simulink model "SWC_APS_type"  (R2021b)
settings: Solver=FixedStepDiscrete  StartTime=0.0  StopTime=10.0  RelTol=1e-3
settings Model: DataDictionary=APPTypes.sldd  Creator=FVT23010  LastModifiedBy=FVT23010
settings DataIOCC: SaveFormat=StructureWithTime
settings OptimizationCC: DefaultParameterBehavior=Inlined  EnhancedBackFolding=on  PassReuseOutputArgsAs=Individual arguments  ZeroExternalMemoryAtStartup=off  ZeroInternalMemoryAtStartup=off  OptimizeBlockOrder=speed  DifferentSizesBufferReuse=on  OptimizationCustomize=off  EfficientTunableParamExpr=on
settings DebuggingCC: ParameterTunabilityLossMsg=error
settings SFSimCC: MATLABDynamicMemAlloc=off
settings RTWCC: Description=AUTOSAR  SystemTargetFile=autosar.tlc  GenCodeOnly=on  TemplateMakefile=ert_default_tmf
settings CodeAppCC: ForceParamTrailComments=on  IgnoreCustomStorageClasses=off  OperatorAnnotations=on  SimulinkDataObjDesc=on  SFDataObjDesc=on  InsertBlockDesc=on
settings STFCustomTargetCC: TargetLangStandard=C99 (ISO)  MultiwordLength=256  ParMdlRefBuildCompliant=on  CompOptLevelCompliant=on  IncludeMdlTerminateFcn=off  CombineOutputUpdateFcns=on  SuppressErrorStatus=on  ERTCustomFileBanners=on  SupportNonFinite=off  SupportComplex=off  SupportContinuousTime=off  SupportNonInlinedSFcns=off  RemoveResetFunc=on  MATLABClassNameForMDSCustomization=Simulink.SoftwareTarget.ERTCustomization  AutosarCompliant=on  GRTInterface=off  UseToolchainInfoCompliant=on  LookupTableObjectStructAxisOrder=2,1,3,4,...  LUTObjectStructOrderEvenSpacing=Size,Table,Breakpoints  SystemTargetFile=autosar.tlc
settings ERTTargetCC: TargetLangStandard=C99 (ISO)  ConcurrentExecutionCompliant=off  IncludeMdlTerminateFcn=off  SuppressErrorStatus=on  SupportNonFinite=off  SupportComplex=off  ModelStepFunctionPrototypeControlCompliant=off  CPPClassGenCompliant=off  AutosarCompliant=on  LookupTableObjectStructAxisOrder=2,1,3,4,...  LUTObjectStructOrderEvenSpacing=Size,Table,Breakpoints  InlinedParameterPlacement=NonHierarchical  ERTCustomFileTemplate=example_file_process.tlc

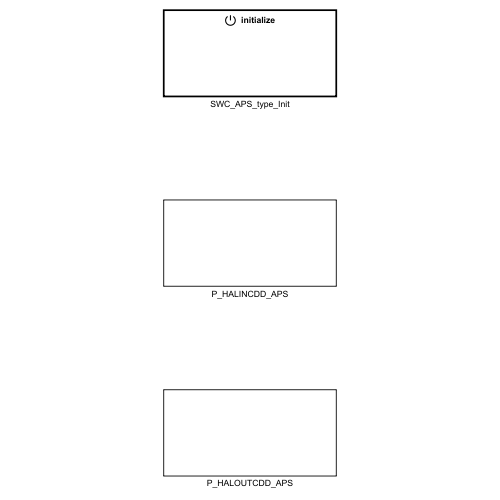
[thumbnail: Simulink's stored preview of the top-level diagram]
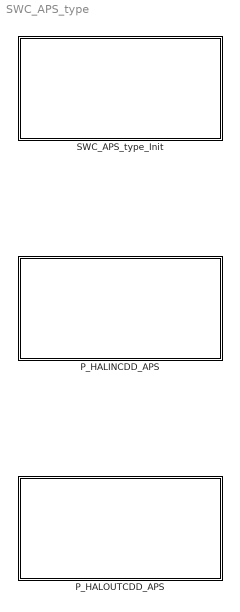
== system SWC_APS_type ==
  P_HALINCDD_APS : Subsystem
  P_HALOUTCDD_APS : Subsystem
  SWC_APS_type_Init : Subsystem

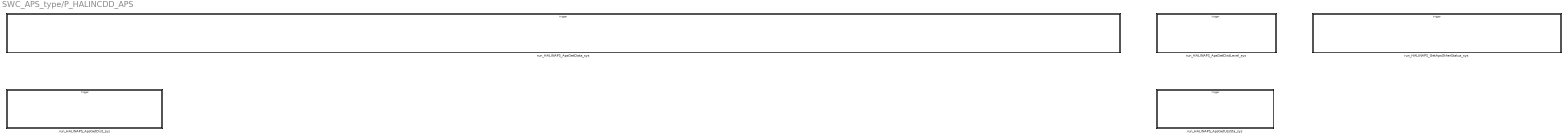
== system SWC_APS_type/P_HALINCDD_APS ==
  run_HALINAPS_ApsGetData_sys : Subsystem
  run_HALINAPS_ApsGetDistLevel_sys : Subsystem
  run_HALINAPS_ApsGetDist_sys : Subsystem
  run_HALINAPS_ApsGetUssSta_sys : Subsystem
  run_HALINAPS_GetApsOtherStatus_sys : Subsystem

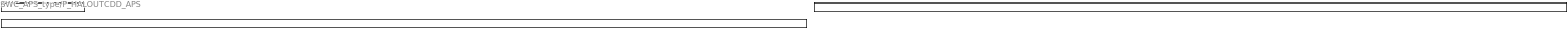
== system SWC_APS_type/P_HALOUTCDD_APS ==
  run_HALOUTAPS_ApsOutput_sys : Subsystem
  run_HALOUTAPS_ApsSetData_sys : Subsystem
  run_HALOUTAPS_ApsSetTimeout_sys : Subsystem

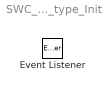
== system SWC_APS_type/SWC_APS_type_Init ==
  Event Listener : EventListener  EventName=reset

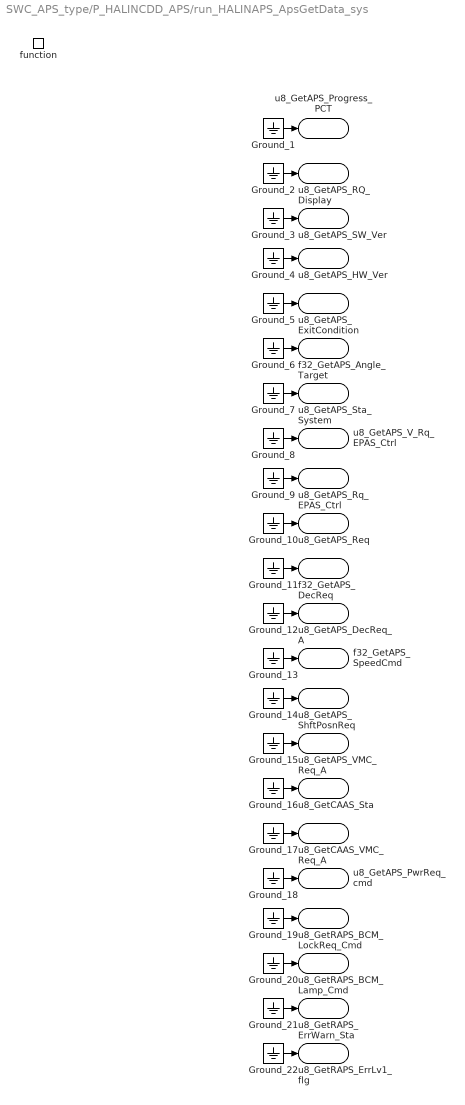
== system SWC_APS_type/P_HALINCDD_APS/run_HALINAPS_ApsGetData_sys ==
  function : TriggerPort  TriggerType=function-call  IsSimulinkFunction=on  FunctionName=run_HALINAPS_ApsGetData  VariantControl=(inherit)
  Ground_{1..22} (22 alike) : Ground
  u8_GetAPS_Progress_PCT : ArgOut  OutDataTypeStr=uint8  ArgumentName=u8_GetAPS_Progress_PCT
  u8_GetAPS_RQ_Display : ArgOut  Port=2  OutDataTypeStr=uint8  ArgumentName=u8_GetAPS_RQ_Display
  u8_GetAPS_SW_Ver : ArgOut  Port=3  OutDataTypeStr=uint8  ArgumentName=u8_GetAPS_SW_Ver
  u8_GetAPS_HW_Ver : ArgOut  Port=4  OutDataTypeStr=uint8  ArgumentName=u8_GetAPS_HW_Ver
  u8_GetAPS_ExitCondition : ArgOut  Port=5  OutDataTypeStr=uint8  ArgumentName=u8_GetAPS_ExitCondition
  f32_GetAPS_Angle_Target : ArgOut  Port=6  OutDataTypeStr=single  ArgumentName=f32_GetAPS_Angle_Target
  u8_GetAPS_Sta_System : ArgOut  Port=7  OutDataTypeStr=uint8  ArgumentName=u8_GetAPS_Sta_System
  u8_GetAPS_V_Rq_EPAS_Ctrl : ArgOut  Port=8  OutDataTypeStr=uint8  ArgumentName=u8_GetAPS_V_Rq_EPAS_Ctrl
  u8_GetAPS_Rq_EPAS_Ctrl : ArgOut  Port=9  OutDataTypeStr=uint8  ArgumentName=u8_GetAPS_Rq_EPAS_Ctrl
  u8_GetAPS_Req : ArgOut  Port=10  OutDataTypeStr=uint8  ArgumentName=u8_GetAPS_Req
  f32_GetAPS_DecReq : ArgOut  Port=11  OutDataTypeStr=single  ArgumentName=f32_GetAPS_DecReq
  u8_GetAPS_DecReq_A : ArgOut  Port=12  OutDataTypeStr=uint8  ArgumentName=u8_GetAPS_DecReq_A
  f32_GetAPS_SpeedCmd : ArgOut  Port=13  OutDataTypeStr=single  ArgumentName=f32_GetAPS_SpeedCmd
  u8_GetAPS_ShftPosnReq : ArgOut  Port=14  OutDataTypeStr=uint8  ArgumentName=u8_GetAPS_ShftPosnReq
  u8_GetAPS_VMC_Req_A : ArgOut  Port=15  OutDataTypeStr=uint8  ArgumentName=u8_GetAPS_VMC_Req_A
  u8_GetCAAS_Sta : ArgOut  Port=16  OutDataTypeStr=uint8  ArgumentName=u8_GetCAAS_Sta
  u8_GetCAAS_VMC_Req_A : ArgOut  Port=17  OutDataTypeStr=uint8  ArgumentName=u8_GetCAAS_VMC_Req_A
  u8_GetAPS_PwrReq_cmd : ArgOut  Port=18  OutDataTypeStr=uint8  ArgumentName=u8_GetAPS_PwrReq_cmd
  u8_GetRAPS_BCM_LockReq_Cmd : ArgOut  Port=19  OutDataTypeStr=uint8  ArgumentName=u8_GetRAPS_BCM_LockReq_Cmd
  u8_GetRAPS_BCM_Lamp_Cmd : ArgOut  Port=20  OutDataTypeStr=uint8  ArgumentName=u8_GetRAPS_BCM_Lamp_Cmd
  u8_GetRAPS_ErrWarn_Sta : ArgOut  Port=21  OutDataTypeStr=uint8  ArgumentName=u8_GetRAPS_ErrWarn_Sta
  u8_GetRAPS_ErrLv1_flg : ArgOut  Port=22  OutDataTypeStr=uint8  ArgumentName=u8_GetRAPS_ErrLv1_flg
  wires:
  Ground_1/1 -> u8_GetAPS_Progress_PCT/1
  Ground_2/1 -> u8_GetAPS_RQ_Display/1
  Ground_3/1 -> u8_GetAPS_SW_Ver/1
  Ground_4/1 -> u8_GetAPS_HW_Ver/1
  Ground_5/1 -> u8_GetAPS_ExitCondition/1
  Ground_6/1 -> f32_GetAPS_Angle_Target/1
  Ground_7/1 -> u8_GetAPS_Sta_System/1
  Ground_8/1 -> u8_GetAPS_V_Rq_EPAS_Ctrl/1
  Ground_9/1 -> u8_GetAPS_Rq_EPAS_Ctrl/1
  Ground_10/1 -> u8_GetAPS_Req/1
  Ground_11/1 -> f32_GetAPS_DecReq/1
  Ground_12/1 -> u8_GetAPS_DecReq_A/1
  Ground_13/1 -> f32_GetAPS_SpeedCmd/1
  Ground_14/1 -> u8_GetAPS_ShftPosnReq/1
  Ground_15/1 -> u8_GetAPS_VMC_Req_A/1
  Ground_16/1 -> u8_GetCAAS_Sta/1
  Ground_17/1 -> u8_GetCAAS_VMC_Req_A/1
  Ground_18/1 -> u8_GetAPS_PwrReq_cmd/1
  Ground_19/1 -> u8_GetRAPS_BCM_LockReq_Cmd/1
  Ground_20/1 -> u8_GetRAPS_BCM_Lamp_Cmd/1
  Ground_21/1 -> u8_GetRAPS_ErrWarn_Sta/1
  Ground_22/1 -> u8_GetRAPS_ErrLv1_flg/1

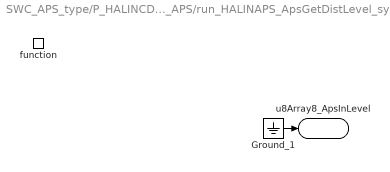
== system SWC_APS_type/P_HALINCDD_APS/run_HALINAPS_ApsGetDistLevel_sys ==
  function : TriggerPort  TriggerType=function-call  IsSimulinkFunction=on  FunctionName=run_HALINAPS_ApsGetDistLevel  VariantControl=(inherit)
  Ground_1 : Ground
  u8Array8_ApsInLevel : ArgOut  OutDataTypeStr=uint8  PortDimensions=8  ArgumentName=u8Array8_ApsInLevel
  wires:
  Ground_1/1 -> u8Array8_ApsInLevel/1

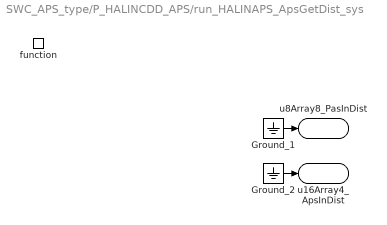
== system SWC_APS_type/P_HALINCDD_APS/run_HALINAPS_ApsGetDist_sys ==
  function : TriggerPort  TriggerType=function-call  IsSimulinkFunction=on  FunctionName=run_HALINAPS_ApsGetDist  VariantControl=(inherit)
  Ground_1 : Ground
  Ground_2 : Ground
  u8Array8_PasInDist : ArgOut  OutDataTypeStr=uint8  PortDimensions=8  ArgumentName=u8Array8_PasInDist
  u16Array4_ApsInDist : ArgOut  Port=2  OutDataTypeStr=uint16  PortDimensions=4  ArgumentName=u16Array4_ApsInDist
  wires:
  Ground_1/1 -> u8Array8_PasInDist/1
  Ground_2/1 -> u16Array4_ApsInDist/1

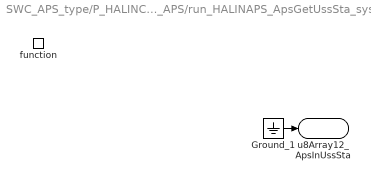
== system SWC_APS_type/P_HALINCDD_APS/run_HALINAPS_ApsGetUssSta_sys ==
  function : TriggerPort  TriggerType=function-call  IsSimulinkFunction=on  FunctionName=run_HALINAPS_ApsGetUssSta  VariantControl=(inherit)
  Ground_1 : Ground
  u8Array12_ApsInUssSta : ArgOut  OutDataTypeStr=uint8  PortDimensions=12  ArgumentName=u8Array12_ApsInUssSta
  wires:
  Ground_1/1 -> u8Array12_ApsInUssSta/1

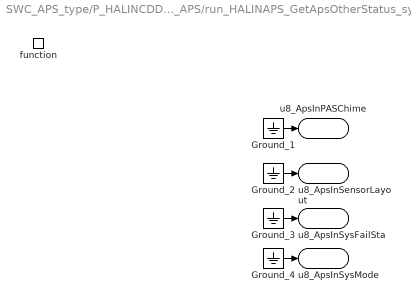
== system SWC_APS_type/P_HALINCDD_APS/run_HALINAPS_GetApsOtherStatus_sys ==
  function : TriggerPort  TriggerType=function-call  IsSimulinkFunction=on  FunctionName=run_HALINAPS_GetApsOtherStatus  VariantControl=(inherit)
  Ground_{1..4} (4 alike) : Ground
  u8_ApsInPASChime : ArgOut  OutDataTypeStr=uint8  ArgumentName=u8_ApsInPASChime
  u8_ApsInSensorLayout : ArgOut  Port=2  OutDataTypeStr=uint8  ArgumentName=u8_ApsInSensorLayout
  u8_ApsInSysFailSta : ArgOut  Port=3  OutDataTypeStr=uint8  ArgumentName=u8_ApsInSysFailSta
  u8_ApsInSysMode : ArgOut  Port=4  OutDataTypeStr=uint8  ArgumentName=u8_ApsInSysMode
  wires:
  Ground_1/1 -> u8_ApsInPASChime/1
  Ground_2/1 -> u8_ApsInSensorLayout/1
  Ground_3/1 -> u8_ApsInSysFailSta/1
  Ground_4/1 -> u8_ApsInSysMode/1

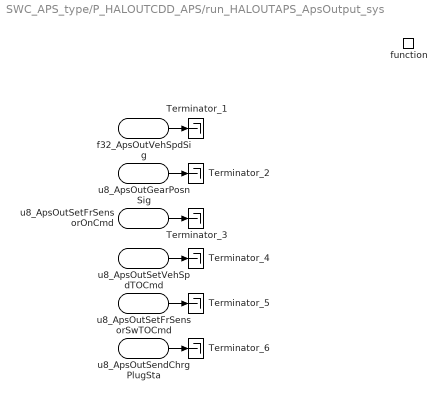
== system SWC_APS_type/P_HALOUTCDD_APS/run_HALOUTAPS_ApsOutput_sys ==
  function : TriggerPort  TriggerType=function-call  IsSimulinkFunction=on  FunctionName=run_HALOUTAPS_ApsOutput  VariantControl=(inherit)
  Terminator_{1..6} (6 alike) : Terminator
  f32_ApsOutVehSpdSig : ArgIn  OutDataTypeStr=single  ArgumentName=f32_ApsOutVehSpdSig
  u8_ApsOutGearPosnSig : ArgIn  Port=2  OutDataTypeStr=uint8  ArgumentName=u8_ApsOutGearPosnSig
  u8_ApsOutSetFrSensorOnCmd : ArgIn  Port=3  OutDataTypeStr=uint8  ArgumentName=u8_ApsOutSetFrSensorOnCmd
  u8_ApsOutSetVehSpdTOCmd : ArgIn  Port=4  OutDataTypeStr=uint8  ArgumentName=u8_ApsOutSetVehSpdTOCmd
  u8_ApsOutSetFrSensorSwTOCmd : ArgIn  Port=5  OutDataTypeStr=uint8  ArgumentName=u8_ApsOutSetFrSensorSwTOCmd
  u8_ApsOutSendChrgPlugSta : ArgIn  Port=6  OutDataTypeStr=uint8  ArgumentName=u8_ApsOutSendChrgPlugSta
  wires:
  f32_ApsOutVehSpdSig/1 -> Terminator_1/1
  u8_ApsOutGearPosnSig/1 -> Terminator_2/1
  u8_ApsOutSetFrSensorOnCmd/1 -> Terminator_3/1
  u8_ApsOutSetVehSpdTOCmd/1 -> Terminator_4/1
  u8_ApsOutSetFrSensorSwTOCmd/1 -> Terminator_5/1
  u8_ApsOutSendChrgPlugSta/1 -> Terminator_6/1

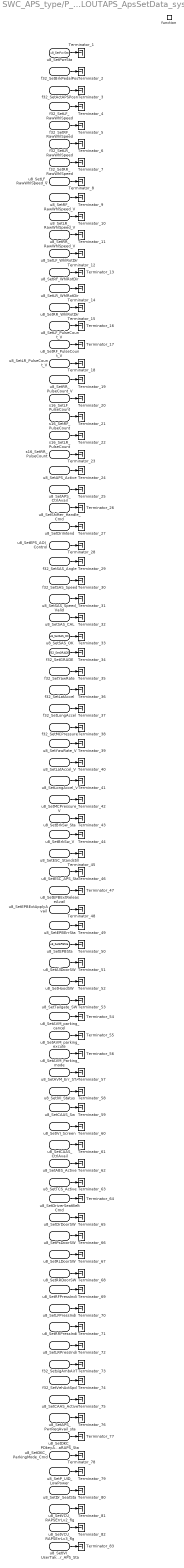
== system SWC_APS_type/P_HALOUTCDD_APS/run_HALOUTAPS_ApsSetData_sys ==
  function : TriggerPort  TriggerType=function-call  IsSimulinkFunction=on  FunctionName=run_HALOUTAPS_ApsSetData  VariantControl=(inherit)
  Terminator_{1..83} (83 alike) : Terminator
  u8_SetPwrSta : ArgIn  OutDataTypeStr=uint8  ArgumentName=u8_SetPwrSta
  f32_SetBrkPedalPos : ArgIn  Port=2  OutDataTypeStr=single  ArgumentName=f32_SetBrkPedalPos
  f32_SetActAPSPosn : ArgIn  Port=3  OutDataTypeStr=single  ArgumentName=f32_SetActAPSPosn
  f32_SetLF_RawWhlSpeed : ArgIn  Port=4  OutDataTypeStr=single  ArgumentName=f32_SetLF_RawWhlSpeed
  f32_SetRF_RawWhlSpeed : ArgIn  Port=5  OutDataTypeStr=single  ArgumentName=f32_SetRF_RawWhlSpeed
  f32_SetLR_RawWhlSpeed : ArgIn  Port=6  OutDataTypeStr=single  ArgumentName=f32_SetLR_RawWhlSpeed
  f32_SetRR_RawWhlSpeed : ArgIn  Port=7  OutDataTypeStr=single  ArgumentName=f32_SetRR_RawWhlSpeed
  u8_SetLF_RawWhlSpeed_V : ArgIn  Port=8  OutDataTypeStr=uint8  ArgumentName=u8_SetLF_RawWhlSpeed_V
  u8_SetRF_RawWhlSpeed_V : ArgIn  Port=9  OutDataTypeStr=uint8  ArgumentName=u8_SetRF_RawWhlSpeed_V
  u8_SetLR_RawWhlSpeed_V : ArgIn  Port=10  OutDataTypeStr=uint8  ArgumentName=u8_SetLR_RawWhlSpeed_V
  u8_SetRR_RawWhlSpeed_V : ArgIn  Port=11  OutDataTypeStr=uint8  ArgumentName=u8_SetRR_RawWhlSpeed_V
  u8_SetLF_WhlRotDir : ArgIn  Port=12  OutDataTypeStr=uint8  ArgumentName=u8_SetLF_WhlRotDir
  u8_SetRF_WhlRotDir : ArgIn  Port=13  OutDataTypeStr=uint8  ArgumentName=u8_SetRF_WhlRotDir
  u8_SetLR_WhlRotDir : ArgIn  Port=14  OutDataTypeStr=uint8  ArgumentName=u8_SetLR_WhlRotDir
  u8_SetRR_WhlRotDir : ArgIn  Port=15  OutDataTypeStr=uint8  ArgumentName=u8_SetRR_WhlRotDir
  u8_SetLF_PulseCount_V : ArgIn  Port=16  OutDataTypeStr=uint8  ArgumentName=u8_SetLF_PulseCount_V
  u8_SetRF_PulseCount_V : ArgIn  Port=17  OutDataTypeStr=uint8  ArgumentName=u8_SetRF_PulseCount_V
  u8_SetLR_PulseCount_V : ArgIn  Port=18  OutDataTypeStr=uint8  ArgumentName=u8_SetLR_PulseCount_V
  u8_SetRR_PulseCount_V : ArgIn  Port=19  OutDataTypeStr=uint8  ArgumentName=u8_SetRR_PulseCount_V
  s16_SetLF_PulseCount : ArgIn  Port=20  OutDataTypeStr=int16  ArgumentName=s16_SetLF_PulseCount
  s16_SetRF_PulseCount : ArgIn  Port=21  OutDataTypeStr=int16  ArgumentName=s16_SetRF_PulseCount
  s16_SetLR_PulseCount : ArgIn  Port=22  OutDataTypeStr=int16  ArgumentName=s16_SetLR_PulseCount
  s16_SetRR_PulseCount : ArgIn  Port=23  OutDataTypeStr=int16  ArgumentName=s16_SetRR_PulseCount
  u8_SetAPS_Active : ArgIn  Port=24  OutDataTypeStr=uint8  ArgumentName=u8_SetAPS_Active
  u8_SetAPS_CtrlAvail : ArgIn  Port=25  OutDataTypeStr=uint8  ArgumentName=u8_SetAPS_CtrlAvail
  u8_SetShifter_Handle_Cmd : ArgIn  Port=26  OutDataTypeStr=uint8  ArgumentName=u8_SetShifter_Handle_Cmd
  u8_SetDriIntend : ArgIn  Port=27  OutDataTypeStr=uint8  ArgumentName=u8_SetDriIntend
  u8_SetEPS_AOI_Control : ArgIn  Port=28  OutDataTypeStr=uint8  ArgumentName=u8_SetEPS_AOI_Control
  f32_SetSAS_Angle : ArgIn  Port=29  OutDataTypeStr=single  ArgumentName=f32_SetSAS_Angle
  f32_SetSAS_Speed : ArgIn  Port=30  OutDataTypeStr=single  ArgumentName=f32_SetSAS_Speed
  u8_SetSAS_Speed_Valid : ArgIn  Port=31  OutDataTypeStr=uint8  ArgumentName=u8_SetSAS_Speed_Valid
  u8_SetSAS_CAL : ArgIn  Port=32  OutDataTypeStr=uint8  ArgumentName=u8_SetSAS_CAL
  u8_SetSAS_OK : ArgIn  Port=33  OutDataTypeStr=uint8  ArgumentName=u8_SetSAS_OK
  f32_SetGRADE : ArgIn  Port=34  OutDataTypeStr=single  ArgumentName=f32_SetGRADE
  f32_SetYawRate : ArgIn  Port=35  OutDataTypeStr=single  ArgumentName=f32_SetYawRate
  f32_SetLatAccel : ArgIn  Port=36  OutDataTypeStr=single  ArgumentName=f32_SetLatAccel
  f32_SetLongAccel : ArgIn  Port=37  OutDataTypeStr=single  ArgumentName=f32_SetLongAccel
  f32_SetMCPressure : ArgIn  Port=38  OutDataTypeStr=single  ArgumentName=f32_SetMCPressure
  u8_SetYawRate_V : ArgIn  Port=39  OutDataTypeStr=uint8  ArgumentName=u8_SetYawRate_V
  u8_SetLatAccel_V : ArgIn  Port=40  OutDataTypeStr=uint8  ArgumentName=u8_SetLatAccel_V
  u8_SetLongAccel_V : ArgIn  Port=41  OutDataTypeStr=uint8  ArgumentName=u8_SetLongAccel_V
  u8_SetMCPressure_V : ArgIn  Port=42  OutDataTypeStr=uint8  ArgumentName=u8_SetMCPressure_V
  u8_SetBrkSw_Sta : ArgIn  Port=43  OutDataTypeStr=uint8  ArgumentName=u8_SetBrkSw_Sta
  u8_SetBrkSw_V : ArgIn  Port=44  OutDataTypeStr=uint8  ArgumentName=u8_SetBrkSw_V
  u8_SetESC_Standstill : ArgIn  Port=45  OutDataTypeStr=uint8  ArgumentName=u8_SetESC_Standstill
  u8_SetESC_APS_Sta : ArgIn  Port=46  OutDataTypeStr=uint8  ArgumentName=u8_SetESC_APS_Sta
  u8_SetEPBExtReleaseAvail : ArgIn  Port=47  OutDataTypeStr=uint8  ArgumentName=u8_SetEPBExtReleaseAvail
  u8_SetEPBExtApplyAvail : ArgIn  Port=48  OutDataTypeStr=uint8  ArgumentName=u8_SetEPBExtApplyAvail
  u8_SetEPBErrSta : ArgIn  Port=49  OutDataTypeStr=uint8  ArgumentName=u8_SetEPBErrSta
  u8_SetEPBSta : ArgIn  Port=50  OutDataTypeStr=uint8  ArgumentName=u8_SetEPBSta
  u8_SetAllDoorSW : ArgIn  Port=51  OutDataTypeStr=uint8  ArgumentName=u8_SetAllDoorSW
  u8_SetHoodSW : ArgIn  Port=52  OutDataTypeStr=uint8  ArgumentName=u8_SetHoodSW
  u8_SetTailgate_SW : ArgIn  Port=53  OutDataTypeStr=uint8  ArgumentName=u8_SetTailgate_SW
  u8_SetAVM_parking_cancel : ArgIn  Port=54  OutDataTypeStr=uint8  ArgumentName=u8_SetAVM_parking_cancel
  u8_SetAVM_parking_excute : ArgIn  Port=55  OutDataTypeStr=uint8  ArgumentName=u8_SetAVM_parking_excute
  u8_SetAVM_Parking_mode : ArgIn  Port=56  OutDataTypeStr=uint8  ArgumentName=u8_SetAVM_Parking_mode
  u8_SetAVM_Err_STA : ArgIn  Port=57  OutDataTypeStr=uint8  ArgumentName=u8_SetAVM_Err_STA
  u8_SetIVI_Status : ArgIn  Port=58  OutDataTypeStr=uint8  ArgumentName=u8_SetIVI_Status
  u8_SetCAAS_Sw : ArgIn  Port=59  OutDataTypeStr=uint8  ArgumentName=u8_SetCAAS_Sw
  u8_SetIVI_Screen : ArgIn  Port=60  OutDataTypeStr=uint8  ArgumentName=u8_SetIVI_Screen
  u8_SetCAAS_CtrlAvail : ArgIn  Port=61  OutDataTypeStr=uint8  ArgumentName=u8_SetCAAS_CtrlAvail
  u8_SetABS_Active : ArgIn  Port=62  OutDataTypeStr=uint8  ArgumentName=u8_SetABS_Active
  u8_SetTCS_Active : ArgIn  Port=63  OutDataTypeStr=uint8  ArgumentName=u8_SetTCS_Active
  u8_SetDriverSeatBeltCmd : ArgIn  Port=64  OutDataTypeStr=uint8  ArgumentName=u8_SetDriverSeatBeltCmd
  u8_SetDrDoorSW : ArgIn  Port=65  OutDataTypeStr=uint8  ArgumentName=u8_SetDrDoorSW
  u8_SetPsDoorSW : ArgIn  Port=66  OutDataTypeStr=uint8  ArgumentName=u8_SetPsDoorSW
  u8_SetRLDoorSW : ArgIn  Port=67  OutDataTypeStr=uint8  ArgumentName=u8_SetRLDoorSW
  u8_SetRRDoorSW : ArgIn  Port=68  OutDataTypeStr=uint8  ArgumentName=u8_SetRRDoorSW
  u8_SetRFPressIndi : ArgIn  Port=69  OutDataTypeStr=uint8  ArgumentName=u8_SetRFPressIndi
  u8_SetLFPressIndi : ArgIn  Port=70  OutDataTypeStr=uint8  ArgumentName=u8_SetLFPressIndi
  u8_SetRRPressIndi : ArgIn  Port=71  OutDataTypeStr=uint8  ArgumentName=u8_SetRRPressIndi
  u8_SetLRPressIndi : ArgIn  Port=72  OutDataTypeStr=uint8  ArgumentName=u8_SetLRPressIndi
  f32_SetsigAmbAirT : ArgIn  Port=73  OutDataTypeStr=single  ArgumentName=f32_SetsigAmbAirT
  f32_SetVehActSpd : ArgIn  Port=74  OutDataTypeStr=single  ArgumentName=f32_SetVehActSpd
  u8_SetCAAS_Active : ArgIn  Port=75  OutDataTypeStr=uint8  ArgumentName=u8_SetCAAS_Active
  u8_SetAPS_PwrReqAvail_sta : ArgIn  Port=76  OutDataTypeStr=uint8  ArgumentName=u8_SetAPS_PwrReqAvail_sta
  u8_SetDKC_PDkeyAreaRAPS_Sta : ArgIn  Port=77  OutDataTypeStr=uint8  ArgumentName=u8_SetDKC_PDkeyAreaRAPS_Sta
  u8_SetDKC_ParkingMode_Cmd : ArgIn  Port=78  OutDataTypeStr=uint8  ArgumentName=u8_SetDKC_ParkingMode_Cmd
  u8_SetP_UID_LowPower : ArgIn  Port=79  OutDataTypeStr=uint8  ArgumentName=u8_SetP_UID_LowPower
  u8_SetDr_SeatSta : ArgIn  Port=80  OutDataTypeStr=uint8  ArgumentName=u8_SetDr_SeatSta
  u8_SetVCU_RAPSErrLv2_flg : ArgIn  Port=81  OutDataTypeStr=uint8  ArgumentName=u8_SetVCU_RAPSErrLv2_flg
  u8_SetVCU_RAPSErrLv3_flg : ArgIn  Port=82  OutDataTypeStr=uint8  ArgumentName=u8_SetVCU_RAPSErrLv3_flg
  u8_SetIVI_UserTakeOver_APS_Sta : ArgIn  Port=83  OutDataTypeStr=uint8  ArgumentName=u8_SetIVI_UserTakeOver_APS_Sta
  wires:
  u8_SetPwrSta/1 -> Terminator_1/1
  f32_SetBrkPedalPos/1 -> Terminator_2/1
  f32_SetActAPSPosn/1 -> Terminator_3/1
  f32_SetLF_RawWhlSpeed/1 -> Terminator_4/1
  f32_SetRF_RawWhlSpeed/1 -> Terminator_5/1
  f32_SetLR_RawWhlSpeed/1 -> Terminator_6/1
  f32_SetRR_RawWhlSpeed/1 -> Terminator_7/1
  u8_SetLF_RawWhlSpeed_V/1 -> Terminator_8/1
  u8_SetRF_RawWhlSpeed_V/1 -> Terminator_9/1
  u8_SetLR_RawWhlSpeed_V/1 -> Terminator_10/1
  u8_SetRR_RawWhlSpeed_V/1 -> Terminator_11/1
  u8_SetLF_WhlRotDir/1 -> Terminator_12/1
  u8_SetRF_WhlRotDir/1 -> Terminator_13/1
  u8_SetLR_WhlRotDir/1 -> Terminator_14/1
  u8_SetRR_WhlRotDir/1 -> Terminator_15/1
  u8_SetLF_PulseCount_V/1 -> Terminator_16/1
  u8_SetRF_PulseCount_V/1 -> Terminator_17/1
  u8_SetLR_PulseCount_V/1 -> Terminator_18/1
  u8_SetRR_PulseCount_V/1 -> Terminator_19/1
  s16_SetLF_PulseCount/1 -> Terminator_20/1
  s16_SetRF_PulseCount/1 -> Terminator_21/1
  s16_SetLR_PulseCount/1 -> Terminator_22/1
  s16_SetRR_PulseCount/1 -> Terminator_23/1
  u8_SetAPS_Active/1 -> Terminator_24/1
  u8_SetAPS_CtrlAvail/1 -> Terminator_25/1
  u8_SetShifter_Handle_Cmd/1 -> Terminator_26/1
  u8_SetDriIntend/1 -> Terminator_27/1
  u8_SetEPS_AOI_Control/1 -> Terminator_28/1
  f32_SetSAS_Angle/1 -> Terminator_29/1
  f32_SetSAS_Speed/1 -> Terminator_30/1
  u8_SetSAS_Speed_Valid/1 -> Terminator_31/1
  u8_SetSAS_CAL/1 -> Terminator_32/1
  u8_SetSAS_OK/1 -> Terminator_33/1
  f32_SetGRADE/1 -> Terminator_34/1
  f32_SetYawRate/1 -> Terminator_35/1
  f32_SetLatAccel/1 -> Terminator_36/1
  f32_SetLongAccel/1 -> Terminator_37/1
  f32_SetMCPressure/1 -> Terminator_38/1
  u8_SetYawRate_V/1 -> Terminator_39/1
  u8_SetLatAccel_V/1 -> Terminator_40/1
  u8_SetLongAccel_V/1 -> Terminator_41/1
  u8_SetMCPressure_V/1 -> Terminator_42/1
  u8_SetBrkSw_Sta/1 -> Terminator_43/1
  u8_SetBrkSw_V/1 -> Terminator_44/1
  u8_SetESC_Standstill/1 -> Terminator_45/1
  u8_SetESC_APS_Sta/1 -> Terminator_46/1
  u8_SetEPBExtReleaseAvail/1 -> Terminator_47/1
  u8_SetEPBExtApplyAvail/1 -> Terminator_48/1
  u8_SetEPBErrSta/1 -> Terminator_49/1
  u8_SetEPBSta/1 -> Terminator_50/1
  u8_SetAllDoorSW/1 -> Terminator_51/1
  u8_SetHoodSW/1 -> Terminator_52/1
  u8_SetTailgate_SW/1 -> Terminator_53/1
  u8_SetAVM_parking_cancel/1 -> Terminator_54/1
  u8_SetAVM_parking_excute/1 -> Terminator_55/1
  u8_SetAVM_Parking_mode/1 -> Terminator_56/1
  u8_SetAVM_Err_STA/1 -> Terminator_57/1
  u8_SetIVI_Status/1 -> Terminator_58/1
  u8_SetCAAS_Sw/1 -> Terminator_59/1
  u8_SetIVI_Screen/1 -> Terminator_60/1
  u8_SetCAAS_CtrlAvail/1 -> Terminator_61/1
  u8_SetABS_Active/1 -> Terminator_62/1
  u8_SetTCS_Active/1 -> Terminator_63/1
  u8_SetDriverSeatBeltCmd/1 -> Terminator_64/1
  u8_SetDrDoorSW/1 -> Terminator_65/1
  u8_SetPsDoorSW/1 -> Terminator_66/1
  u8_SetRLDoorSW/1 -> Terminator_67/1
  u8_SetRRDoorSW/1 -> Terminator_68/1
  u8_SetRFPressIndi/1 -> Terminator_69/1
  u8_SetLFPressIndi/1 -> Terminator_70/1
  u8_SetRRPressIndi/1 -> Terminator_71/1
  u8_SetLRPressIndi/1 -> Terminator_72/1
  f32_SetsigAmbAirT/1 -> Terminator_73/1
  f32_SetVehActSpd/1 -> Terminator_74/1
  u8_SetCAAS_Active/1 -> Terminator_75/1
  u8_SetAPS_PwrReqAvail_sta/1 -> Terminator_76/1
  u8_SetDKC_PDkeyAreaRAPS_Sta/1 -> Terminator_77/1
  u8_SetDKC_ParkingMode_Cmd/1 -> Terminator_78/1
  u8_SetP_UID_LowPower/1 -> Terminator_79/1
  u8_SetDr_SeatSta/1 -> Terminator_80/1
  u8_SetVCU_RAPSErrLv2_flg/1 -> Terminator_81/1
  u8_SetVCU_RAPSErrLv3_flg/1 -> Terminator_82/1
  u8_SetIVI_UserTakeOver_APS_Sta/1 -> Terminator_83/1

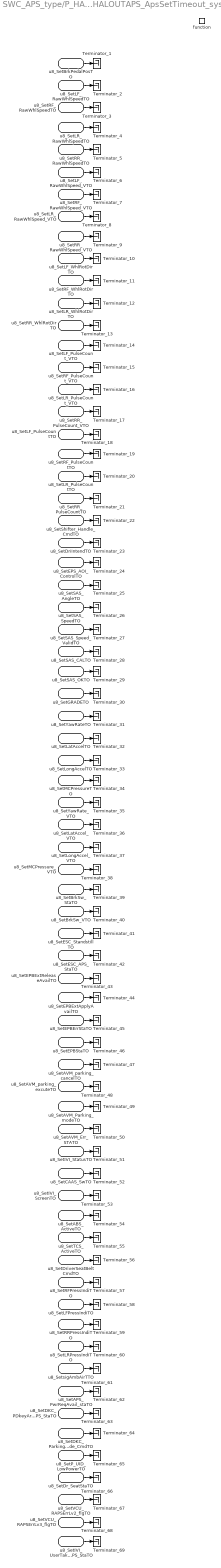
== system SWC_APS_type/P_HALOUTCDD_APS/run_HALOUTAPS_ApsSetTimeout_sys ==
  function : TriggerPort  TriggerType=function-call  IsSimulinkFunction=on  FunctionName=run_HALOUTAPS_ApsSetTimeout  VariantControl=(inherit)
  Terminator_{1..69} (69 alike) : Terminator
  u8_SetBrkPedalPosTO : ArgIn  OutDataTypeStr=uint8  ArgumentName=u8_SetBrkPedalPosTO
  u8_SetLF_RawWhlSpeedTO : ArgIn  Port=2  OutDataTypeStr=uint8  ArgumentName=u8_SetLF_RawWhlSpeedTO
  u8_SetRF_RawWhlSpeedTO : ArgIn  Port=3  OutDataTypeStr=uint8  ArgumentName=u8_SetRF_RawWhlSpeedTO
  u8_SetLR_RawWhlSpeedTO : ArgIn  Port=4  OutDataTypeStr=uint8  ArgumentName=u8_SetLR_RawWhlSpeedTO
  u8_SetRR_RawWhlSpeedTO : ArgIn  Port=5  OutDataTypeStr=uint8  ArgumentName=u8_SetRR_RawWhlSpeedTO
  u8_SetLF_RawWhlSpeed_VTO : ArgIn  Port=6  OutDataTypeStr=uint8  ArgumentName=u8_SetLF_RawWhlSpeed_VTO
  u8_SetRF_RawWhlSpeed_VTO : ArgIn  Port=7  OutDataTypeStr=uint8  ArgumentName=u8_SetRF_RawWhlSpeed_VTO
  u8_SetLR_RawWhlSpeed_VTO : ArgIn  Port=8  OutDataTypeStr=uint8  ArgumentName=u8_SetLR_RawWhlSpeed_VTO
  u8_SetRR_RawWhlSpeed_VTO : ArgIn  Port=9  OutDataTypeStr=uint8  ArgumentName=u8_SetRR_RawWhlSpeed_VTO
  u8_SetLF_WhlRotDirTO : ArgIn  Port=10  OutDataTypeStr=uint8  ArgumentName=u8_SetLF_WhlRotDirTO
  u8_SetRF_WhlRotDirTO : ArgIn  Port=11  OutDataTypeStr=uint8  ArgumentName=u8_SetRF_WhlRotDirTO
  u8_SetLR_WhlRotDirTO : ArgIn  Port=12  OutDataTypeStr=uint8  ArgumentName=u8_SetLR_WhlRotDirTO
  u8_SetRR_WhlRotDirTO : ArgIn  Port=13  OutDataTypeStr=uint8  ArgumentName=u8_SetRR_WhlRotDirTO
  u8_SetLF_PulseCount_VTO : ArgIn  Port=14  OutDataTypeStr=uint8  ArgumentName=u8_SetLF_PulseCount_VTO
  u8_SetRF_PulseCount_VTO : ArgIn  Port=15  OutDataTypeStr=uint8  ArgumentName=u8_SetRF_PulseCount_VTO
  u8_SetLR_PulseCount_VTO : ArgIn  Port=16  OutDataTypeStr=uint8  ArgumentName=u8_SetLR_PulseCount_VTO
  u8_SetRR_PulseCount_VTO : ArgIn  Port=17  OutDataTypeStr=uint8  ArgumentName=u8_SetRR_PulseCount_VTO
  u8_SetLF_PulseCountTO : ArgIn  Port=18  OutDataTypeStr=uint8  ArgumentName=u8_SetLF_PulseCountTO
  u8_SetRF_PulseCountTO : ArgIn  Port=19  OutDataTypeStr=uint8  ArgumentName=u8_SetRF_PulseCountTO
  u8_SetLR_PulseCountTO : ArgIn  Port=20  OutDataTypeStr=uint8  ArgumentName=u8_SetLR_PulseCountTO
  u8_SetRR_PulseCountTO : ArgIn  Port=21  OutDataTypeStr=uint8  ArgumentName=u8_SetRR_PulseCountTO
  u8_SetShifter_Handle_CmdTO : ArgIn  Port=22  OutDataTypeStr=uint8  ArgumentName=u8_SetShifter_Handle_CmdTO
  u8_SetDriIntendTO : ArgIn  Port=23  OutDataTypeStr=uint8  ArgumentName=u8_SetDriIntendTO
  u8_SetEPS_AOI_ControlTO : ArgIn  Port=24  OutDataTypeStr=uint8  ArgumentName=u8_SetEPS_AOI_ControlTO
  u8_SetSAS_AngleTO : ArgIn  Port=25  OutDataTypeStr=uint8  ArgumentName=u8_SetSAS_AngleTO
  u8_SetSAS_SpeedTO : ArgIn  Port=26  OutDataTypeStr=uint8  ArgumentName=u8_SetSAS_SpeedTO
  u8_SetSAS_Speed_ValidTO : ArgIn  Port=27  OutDataTypeStr=uint8  ArgumentName=u8_SetSAS_Speed_ValidTO
  u8_SetSAS_CALTO : ArgIn  Port=28  OutDataTypeStr=uint8  ArgumentName=u8_SetSAS_CALTO
  u8_SetSAS_OKTO : ArgIn  Port=29  OutDataTypeStr=uint8  ArgumentName=u8_SetSAS_OKTO
  u8_SetGRADETO : ArgIn  Port=30  OutDataTypeStr=uint8  ArgumentName=u8_SetGRADETO
  u8_SetYawRateTO : ArgIn  Port=31  OutDataTypeStr=uint8  ArgumentName=u8_SetYawRateTO
  u8_SetLatAccelTO : ArgIn  Port=32  OutDataTypeStr=uint8  ArgumentName=u8_SetLatAccelTO
  u8_SetLongAccelTO : ArgIn  Port=33  OutDataTypeStr=uint8  ArgumentName=u8_SetLongAccelTO
  u8_SetMCPressureTO : ArgIn  Port=34  OutDataTypeStr=uint8  ArgumentName=u8_SetMCPressureTO
  u8_SetYawRate_VTO : ArgIn  Port=35  OutDataTypeStr=uint8  ArgumentName=u8_SetYawRate_VTO
  u8_SetLatAccel_VTO : ArgIn  Port=36  OutDataTypeStr=uint8  ArgumentName=u8_SetLatAccel_VTO
  u8_SetLongAccel_VTO : ArgIn  Port=37  OutDataTypeStr=uint8  ArgumentName=u8_SetLongAccel_VTO
  u8_SetMCPressure_VTO : ArgIn  Port=38  OutDataTypeStr=uint8  ArgumentName=u8_SetMCPressure_VTO
  u8_SetBrkSw_StaTO : ArgIn  Port=39  OutDataTypeStr=uint8  ArgumentName=u8_SetBrkSw_StaTO
  u8_SetBrkSw_VTO : ArgIn  Port=40  OutDataTypeStr=uint8  ArgumentName=u8_SetBrkSw_VTO
  u8_SetESC_StandstillTO : ArgIn  Port=41  OutDataTypeStr=uint8  ArgumentName=u8_SetESC_StandstillTO
  u8_SetESC_APS_StaTO : ArgIn  Port=42  OutDataTypeStr=uint8  ArgumentName=u8_SetESC_APS_StaTO
  u8_SetEPBExtReleaseAvailTO : ArgIn  Port=43  OutDataTypeStr=uint8  ArgumentName=u8_SetEPBExtReleaseAvailTO
  u8_SetEPBExtApplyAvailTO : ArgIn  Port=44  OutDataTypeStr=uint8  ArgumentName=u8_SetEPBExtApplyAvailTO
  u8_SetEPBErrStaTO : ArgIn  Port=45  OutDataTypeStr=uint8  ArgumentName=u8_SetEPBErrStaTO
  u8_SetEPBStaTO : ArgIn  Port=46  OutDataTypeStr=uint8  ArgumentName=u8_SetEPBStaTO
  u8_SetAVM_parking_cancelTO : ArgIn  Port=47  OutDataTypeStr=uint8  ArgumentName=u8_SetAVM_parking_cancelTO
  u8_SetAVM_parking_excuteTO : ArgIn  Port=48  OutDataTypeStr=uint8  ArgumentName=u8_SetAVM_parking_excuteTO
  u8_SetAVM_Parking_modeTO : ArgIn  Port=49  OutDataTypeStr=uint8  ArgumentName=u8_SetAVM_Parking_modeTO
  u8_SetAVM_Err_STATO : ArgIn  Port=50  OutDataTypeStr=uint8  ArgumentName=u8_SetAVM_Err_STATO
  u8_SetIVI_StatusTO : ArgIn  Port=51  OutDataTypeStr=uint8  ArgumentName=u8_SetIVI_StatusTO
  u8_SetCAAS_SwTO : ArgIn  Port=52  OutDataTypeStr=uint8  ArgumentName=u8_SetCAAS_SwTO
  u8_SetIVI_ScreenTO : ArgIn  Port=53  OutDataTypeStr=uint8  ArgumentName=u8_SetIVI_ScreenTO
  u8_SetABS_ActiveTO : ArgIn  Port=54  OutDataTypeStr=uint8  ArgumentName=u8_SetABS_ActiveTO
  u8_SetTCS_ActiveTO : ArgIn  Port=55  OutDataTypeStr=uint8  ArgumentName=u8_SetTCS_ActiveTO
  u8_SetDriverSeatBeltCmdTO : ArgIn  Port=56  OutDataTypeStr=uint8  ArgumentName=u8_SetDriverSeatBeltCmdTO
  u8_SetRFPressIndiTO : ArgIn  Port=57  OutDataTypeStr=uint8  ArgumentName=u8_SetRFPressIndiTO
  u8_SetLFPressIndiTO : ArgIn  Port=58  OutDataTypeStr=uint8  ArgumentName=u8_SetLFPressIndiTO
  u8_SetRRPressIndiTO : ArgIn  Port=59  OutDataTypeStr=uint8  ArgumentName=u8_SetRRPressIndiTO
  u8_SetLRPressIndiTO : ArgIn  Port=60  OutDataTypeStr=uint8  ArgumentName=u8_SetLRPressIndiTO
  u8_SetsigAmbAirTTO : ArgIn  Port=61  OutDataTypeStr=uint8  ArgumentName=u8_SetsigAmbAirTTO
  u8_SetAPS_PwrReqAvail_staTO : ArgIn  Port=62  OutDataTypeStr=uint8  ArgumentName=u8_SetAPS_PwrReqAvail_staTO
  u8_SetDKC_PDkeyAreaRAPS_StaTO : ArgIn  Port=63  OutDataTypeStr=uint8  ArgumentName=u8_SetDKC_PDkeyAreaRAPS_StaTO
  u8_SetDKC_ParkingMode_CmdTO : ArgIn  Port=64  OutDataTypeStr=uint8  ArgumentName=u8_SetDKC_ParkingMode_CmdTO
  u8_SetP_UID_LowPowerTO : ArgIn  Port=65  OutDataTypeStr=uint8  ArgumentName=u8_SetP_UID_LowPowerTO
  u8_SetDr_SeatStaTO : ArgIn  Port=66  OutDataTypeStr=uint8  ArgumentName=u8_SetDr_SeatStaTO
  u8_SetVCU_RAPSErrLv2_flgTO : ArgIn  Port=67  OutDataTypeStr=uint8  ArgumentName=u8_SetVCU_RAPSErrLv2_flgTO
  u8_SetVCU_RAPSErrLv3_flgTO : ArgIn  Port=68  OutDataTypeStr=uint8  ArgumentName=u8_SetVCU_RAPSErrLv3_flgTO
  u8_SetIVI_UserTakeOver_APS_StaTO : ArgIn  Port=69  OutDataTypeStr=uint8  ArgumentName=u8_SetIVI_UserTakeOver_APS_StaTO
  wires:
  u8_SetBrkPedalPosTO/1 -> Terminator_1/1
  u8_SetLF_RawWhlSpeedTO/1 -> Terminator_2/1
  u8_SetRF_RawWhlSpeedTO/1 -> Terminator_3/1
  u8_SetLR_RawWhlSpeedTO/1 -> Terminator_4/1
  u8_SetRR_RawWhlSpeedTO/1 -> Terminator_5/1
  u8_SetLF_RawWhlSpeed_VTO/1 -> Terminator_6/1
  u8_SetRF_RawWhlSpeed_VTO/1 -> Terminator_7/1
  u8_SetLR_RawWhlSpeed_VTO/1 -> Terminator_8/1
  u8_SetRR_RawWhlSpeed_VTO/1 -> Terminator_9/1
  u8_SetLF_WhlRotDirTO/1 -> Terminator_10/1
  u8_SetRF_WhlRotDirTO/1 -> Terminator_11/1
  u8_SetLR_WhlRotDirTO/1 -> Terminator_12/1
  u8_SetRR_WhlRotDirTO/1 -> Terminator_13/1
  u8_SetLF_PulseCount_VTO/1 -> Terminator_14/1
  u8_SetRF_PulseCount_VTO/1 -> Terminator_15/1
  u8_SetLR_PulseCount_VTO/1 -> Terminator_16/1
  u8_SetRR_PulseCount_VTO/1 -> Terminator_17/1
  u8_SetLF_PulseCountTO/1 -> Terminator_18/1
  u8_SetRF_PulseCountTO/1 -> Terminator_19/1
  u8_SetLR_PulseCountTO/1 -> Terminator_20/1
  u8_SetRR_PulseCountTO/1 -> Terminator_21/1
  u8_SetShifter_Handle_CmdTO/1 -> Terminator_22/1
  u8_SetDriIntendTO/1 -> Terminator_23/1
  u8_SetEPS_AOI_ControlTO/1 -> Terminator_24/1
  u8_SetSAS_AngleTO/1 -> Terminator_25/1
  u8_SetSAS_SpeedTO/1 -> Terminator_26/1
  u8_SetSAS_Speed_ValidTO/1 -> Terminator_27/1
  u8_SetSAS_CALTO/1 -> Terminator_28/1
  u8_SetSAS_OKTO/1 -> Terminator_29/1
  u8_SetGRADETO/1 -> Terminator_30/1
  u8_SetYawRateTO/1 -> Terminator_31/1
  u8_SetLatAccelTO/1 -> Terminator_32/1
  u8_SetLongAccelTO/1 -> Terminator_33/1
  u8_SetMCPressureTO/1 -> Terminator_34/1
  u8_SetYawRate_VTO/1 -> Terminator_35/1
  u8_SetLatAccel_VTO/1 -> Terminator_36/1
  u8_SetLongAccel_VTO/1 -> Terminator_37/1
  u8_SetMCPressure_VTO/1 -> Terminator_38/1
  u8_SetBrkSw_StaTO/1 -> Terminator_39/1
  u8_SetBrkSw_VTO/1 -> Terminator_40/1
  u8_SetESC_StandstillTO/1 -> Terminator_41/1
  u8_SetESC_APS_StaTO/1 -> Terminator_42/1
  u8_SetEPBExtReleaseAvailTO/1 -> Terminator_43/1
  u8_SetEPBExtApplyAvailTO/1 -> Terminator_44/1
  u8_SetEPBErrStaTO/1 -> Terminator_45/1
  u8_SetEPBStaTO/1 -> Terminator_46/1
  u8_SetAVM_parking_cancelTO/1 -> Terminator_47/1
  u8_SetAVM_parking_excuteTO/1 -> Terminator_48/1
  u8_SetAVM_Parking_modeTO/1 -> Terminator_49/1
  u8_SetAVM_Err_STATO/1 -> Terminator_50/1
  u8_SetIVI_StatusTO/1 -> Terminator_51/1
  u8_SetCAAS_SwTO/1 -> Terminator_52/1
  u8_SetIVI_ScreenTO/1 -> Terminator_53/1
  u8_SetABS_ActiveTO/1 -> Terminator_54/1
  u8_SetTCS_ActiveTO/1 -> Terminator_55/1
  u8_SetDriverSeatBeltCmdTO/1 -> Terminator_56/1
  u8_SetRFPressIndiTO/1 -> Terminator_57/1
  u8_SetLFPressIndiTO/1 -> Terminator_58/1
  u8_SetRRPressIndiTO/1 -> Terminator_59/1
  u8_SetLRPressIndiTO/1 -> Terminator_60/1
  u8_SetsigAmbAirTTO/1 -> Terminator_61/1
  u8_SetAPS_PwrReqAvail_staTO/1 -> Terminator_62/1
  u8_SetDKC_PDkeyAreaRAPS_StaTO/1 -> Terminator_63/1
  u8_SetDKC_ParkingMode_CmdTO/1 -> Terminator_64/1
  u8_SetP_UID_LowPowerTO/1 -> Terminator_65/1
  u8_SetDr_SeatStaTO/1 -> Terminator_66/1
  u8_SetVCU_RAPSErrLv2_flgTO/1 -> Terminator_67/1
  u8_SetVCU_RAPSErrLv3_flgTO/1 -> Terminator_68/1
  u8_SetIVI_UserTakeOver_APS_StaTO/1 -> Terminator_69/1
